simulink model "model_ex2_FUNCIONA_BIEN"  (R2019b)
settings: Solver=VariableStepDiscrete  StartTime=0.0  StopTime=100.0  RelTol=1e-3
values from neighbouring files (symbols this model uses):
  th_0 = input(ask_th)    [simData2.m]
  Ts = Ts * 10.^-3    (= 0.0001)    [simData2.m]
  x_0 = input(ask_x)    [simData2.m]
  y_0 = input(ask_y)    [simData2.m]
undefined symbols (not defined in the file or in its folder): DiscIntNeverNeededParam, sigbuilder_block
libraries: simulink x1
settings Model: Creator=Laura  LastModifiedBy=Laura
settings DataIOCC: SaveFormat=StructureWithTime  ReturnWorkspaceOutputs=off

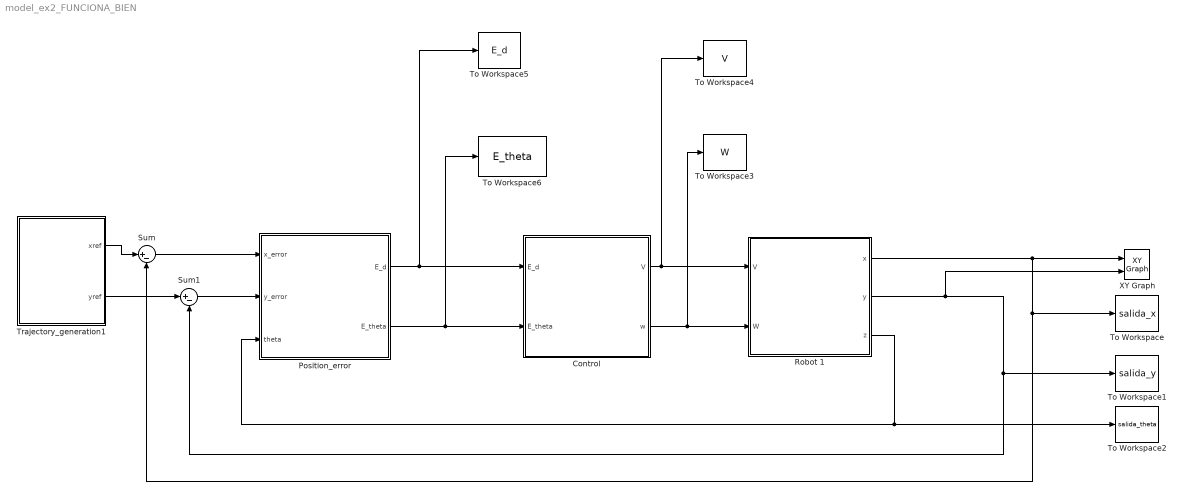
== system model_ex2_FUNCIONA_BIEN ==
  Control : Subsystem
  "Position_error " : Subsystem
  Robot 1 : Subsystem
  Sum : Sum  Inputs=|+-
  Sum1 : Sum  Inputs=|+-
  To Workspace : ToWorkspace  VariableName=salida_x  SaveFormat=Structure With Time  SampleTime=-1
      settings: Save2DSignal=2-D array (concatenate along first dimension)
  To Workspace1 : ToWorkspace  VariableName=salida_y  SaveFormat=Structure With Time  SampleTime=-1
      settings: Save2DSignal=2-D array (concatenate along first dimension)
  To Workspace2 : ToWorkspace  VariableName=salida_theta  SaveFormat=Structure With Time  SampleTime=-1
      settings: Save2DSignal=2-D array (concatenate along first dimension)
  To Workspace3 : ToWorkspace  VariableName=W  SaveFormat=Structure With Time  SampleTime=-1
      settings: Save2DSignal=2-D array (concatenate along first dimension)
  To Workspace4 : ToWorkspace  VariableName=V  SaveFormat=Structure With Time  SampleTime=-1
      settings: Save2DSignal=2-D array (concatenate along first dimension)
  To Workspace5 : ToWorkspace  VariableName=E_d  SaveFormat=Structure With Time  SampleTime=-1
      settings: Save2DSignal=2-D array (concatenate along first dimension)
  To Workspace6 : ToWorkspace  VariableName=E_theta  SaveFormat=Structure With Time  SampleTime=-1
      settings: Save2DSignal=2-D array (concatenate along first dimension)
  Trajectory_generation1 : Subsystem
  XY Graph : simulink/Sinks/XY Graph  xmin=-5  xmax=5  ymin=-5  ymax=5  st=-1
  wires:
  Robot 1/2(y) -> XY Graph/2, Sum1/2, To Workspace1/1
  Control/1(V) -> Robot 1/1("V "), To Workspace4/1
  Control/2(w) -> Robot 1/2("W "), To Workspace3/1
  "Position_error "/1(E_d) -> Control/1(E_d), To Workspace5/1
  Sum/1 -> "Position_error "/1("x_error ")
  "Position_error "/2(E_theta) -> Control/2(E_theta), To Workspace6/1
  Robot 1/1(x) -> XY Graph/1, Sum/2, To Workspace/1
  Robot 1/3(z) -> "Position_error "/3("theta "), To Workspace2/1
  Sum1/1 -> "Position_error "/2("y_error ")
  Trajectory_generation1/1(xref) -> Sum/1
  Trajectory_generation1/2(yref) -> Sum1/1

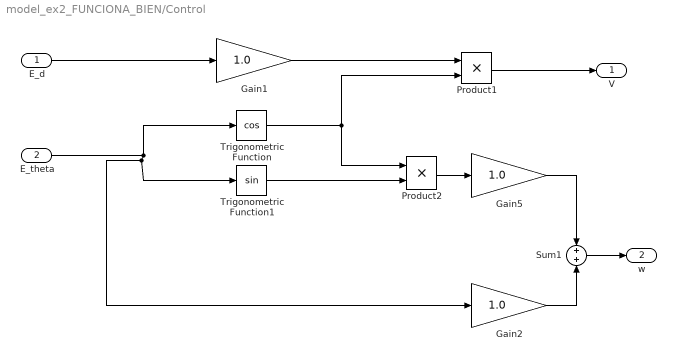
== system model_ex2_FUNCIONA_BIEN/Control ==
  E_d : Inport
  E_theta : Inport  Port=2
  Gain1 : Gain  Gain=1.0
  Gain2 : Gain  Gain=1.0
  Gain5 : Gain  Gain=1.0
  Product1 : Product
  Product2 : Product
  Sum1 : Sum
  Trigonometric Function : Trigonometry  Operator=cos
  Trigonometric Function1 : Trigonometry
  V : Outport  VectorParamsAs1DForOutWhenUnconnected=off
  w : Outport  Port=2  VectorParamsAs1DForOutWhenUnconnected=off
  wires:
  Sum1/1 -> w/1
  Gain2/1 -> Sum1/2
  Gain5/1 -> Sum1/1
  Gain1/1 -> Product1/1
  Product2/1 -> Gain5/1
  Trigonometric Function1/1 -> Product2/2
  Product1/1 -> V/1
  Trigonometric Function/1 -> Product2/1, Product1/2
  E_d/1 -> Gain1/1
  E_theta/1 -> Gain2/1, Trigonometric Function1/1, Trigonometric Function/1

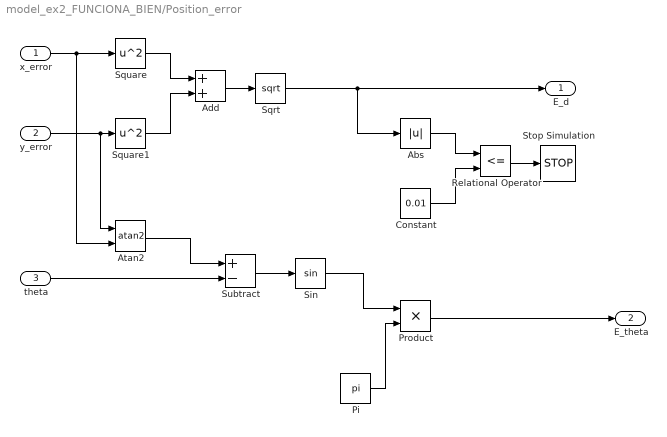
== system model_ex2_FUNCIONA_BIEN/Position_error  ==
  "x_error " : Inport
  "y_error " : Inport  Port=2
  "theta " : Inport  Port=3
  Abs : Abs
  Add : Sum
  Atan2 : Trigonometry  Operator=atan2
  Constant : Constant  Value=0.01
  Pi : Constant  Value=pi  OutDataTypeStr=Inherit: Inherit via back propagation
  Product : Product
  Relational Operator : RelationalOperator  Operator=<=  OutDataTypeStr=boolean  RndMeth=Simplest
  Sin : Trigonometry
  Sqrt : Sqrt  SaturateOnIntegerOverflow=on
  Square : Math  Operator=square  SignedPower=off  SaturateOnIntegerOverflow=on
  Square1 : Math  Operator=square  SignedPower=off  SaturateOnIntegerOverflow=on
  Stop Simulation : Stop
  Subtract : Sum  Inputs=+-
  E_d : Outport
  E_theta : Outport  Port=2
  wires:
  Abs/1 -> Relational Operator/1
  Constant/1 -> Relational Operator/2
  Relational Operator/1 -> Stop Simulation/1
  "x_error "/1 -> Atan2/2, Square/1
  "y_error "/1 -> Atan2/1, Square1/1
  Square/1 -> Add/1
  Square1/1 -> Add/2
  Add/1 -> Sqrt/1
  Atan2/1 -> Subtract/1
  "theta "/1 -> Subtract/2
  Sqrt/1 -> E_d/1, Abs/1
  Subtract/1 -> Sin/1
  Sin/1 -> Product/1
  Pi/1 -> Product/2
  Product/1 -> E_theta/1

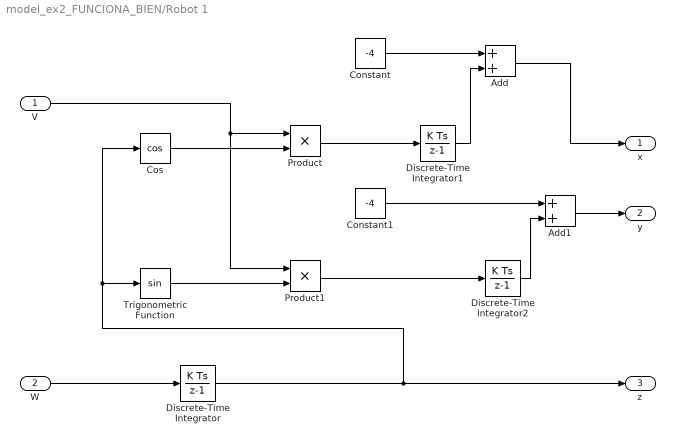
== system model_ex2_FUNCIONA_BIEN/Robot 1 ==
  "V " : Inport
  "W " : Inport  Port=2
  Add : Sum
  Add1 : Sum
  Constant : Constant  Value=-4
  Constant1 : Constant  Value=-4
  Cos : Trigonometry  Operator=cos
  Discrete-Time Integrator : DiscreteIntegrator  InitialCondition=th_0  SampleTime=-1  ICPrevOutput=DiscIntNeverNeededParam  ICPrevScaledInput=DiscIntNeverNeededParam
  Discrete-Time Integrator1 : DiscreteIntegrator  InitialCondition=x_0  SampleTime=-1  ICPrevOutput=DiscIntNeverNeededParam  ICPrevScaledInput=DiscIntNeverNeededParam
  Discrete-Time Integrator2 : DiscreteIntegrator  InitialCondition=y_0  SampleTime=-1  ICPrevOutput=DiscIntNeverNeededParam  ICPrevScaledInput=DiscIntNeverNeededParam
  Product : Product
  Product1 : Product
  Trigonometric Function : Trigonometry
  x : Outport
  y : Outport  Port=2
  z : Outport  Port=3
  wires:
  Product/1 -> Discrete-Time Integrator1/1
  Trigonometric Function/1 -> Product1/2
  Discrete-Time Integrator/1 -> Cos/1, Trigonometric Function/1, z/1
  "W "/1 -> Discrete-Time Integrator/1
  Product1/1 -> Discrete-Time Integrator2/1
  Cos/1 -> Product/2
  "V "/1 -> Product1/1, Product/1
  Discrete-Time Integrator1/1 -> Add/2
  Constant/1 -> Add/1
  Add/1 -> x/1
  Constant1/1 -> Add1/1
  Discrete-Time Integrator2/1 -> Add1/2
  Add1/1 -> y/1

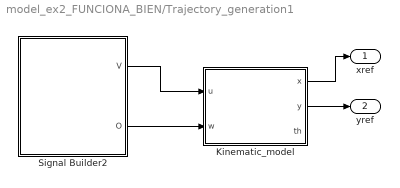
== system model_ex2_FUNCIONA_BIEN/Trajectory_generation1 ==
  Kinematic_model : Subsystem
  Signal Builder2 : Subsystem  Tag=STV Subsys  LoadFcn=sigbuilder_block('load');  StartFcn=sigbuilder_block('start');  StopFcn=sigbuilder_block('stop');  ClipboardFcn=sigbuilder_block('clipboard');  mask(Sigbuilder block){tuvar=[0:10]}
      mask help: Sigbuilder GUI
      mask init:
      | if ~strcmp(get_param(bdroot(gcbh),'SimulationStatus'),'stopped') tuvar = sigbuilder_block('maskInit'); end
      settings: CopyFcn=sigbuilder_block('copy');  DeleteFcn=sigbuilder_block('delete');  ModelCloseFcn=sigbuilder_block('modelClose');  PreSaveFcn=sigbuilder_block('preSave');  PauseFcn=sigbuilder_block('pause')  ContinueFcn=sigbuilder_block('continue')  NameChangeFcn=sigbuilder_block('namechange');  OpenFcn=sigbuilder_block('open',[60 82.4 534.4 508 ]);  CloseFcn=sigbuilder_block('close');
      mask Display: plot(0, 0, 100, 100,[2, 2, 32, 32, 2], [68, 8, 8, 68, 68],[32, 2], [38, 38], [32, 19, 2],[53, 60, 44], [32, 17, 17, 2],[16, 16, 31, 31]);txt = getActiveGroup(gcbh);text(2, 100, txt,'verticalAlignment', 'top');
  xref : Outport  VectorParamsAs1DForOutWhenUnconnected=off
  yref : Outport  Port=2  VectorParamsAs1DForOutWhenUnconnected=off
  wires:
  Signal Builder2/1(V) -> Kinematic_model/1(u)
  Signal Builder2/2(O) -> Kinematic_model/2(w)
  Kinematic_model/1(x) -> xref/1
  Kinematic_model/2(y) -> yref/1

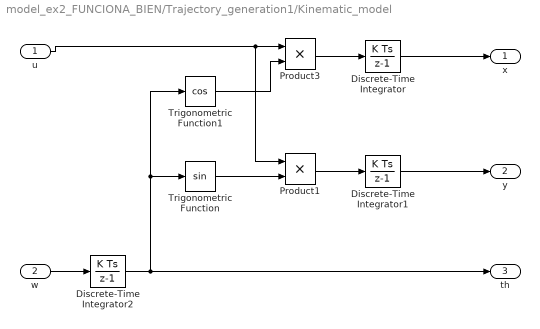
== system model_ex2_FUNCIONA_BIEN/Trajectory_generation1/Kinematic_model ==
  u : Inport
  w : Inport  Port=2
  Discrete-Time Integrator : DiscreteIntegrator  InitialCondition=x_0  SampleTime=Ts  ICPrevOutput=DiscIntNeverNeededParam  ICPrevScaledInput=DiscIntNeverNeededParam
  Discrete-Time Integrator1 : DiscreteIntegrator  InitialCondition=y_0  SampleTime=Ts  ICPrevOutput=DiscIntNeverNeededParam  ICPrevScaledInput=DiscIntNeverNeededParam
  Discrete-Time Integrator2 : DiscreteIntegrator  InitialCondition=th_0  SampleTime=Ts  ICPrevOutput=DiscIntNeverNeededParam  ICPrevScaledInput=DiscIntNeverNeededParam
  Product1 : Product
  Product3 : Product
  Trigonometric Function : Trigonometry
  Trigonometric Function1 : Trigonometry  Operator=cos
  x : Outport  VectorParamsAs1DForOutWhenUnconnected=off
  y : Outport  Port=2  VectorParamsAs1DForOutWhenUnconnected=off
  th : Outport  Port=3  VectorParamsAs1DForOutWhenUnconnected=off
  wires:
  Discrete-Time Integrator2/1 -> Trigonometric Function1/1, Trigonometric Function/1, th/1
  Product1/1 -> Discrete-Time Integrator1/1
  Product3/1 -> Discrete-Time Integrator/1
  w/1 -> Discrete-Time Integrator2/1
  Trigonometric Function/1 -> Product1/2
  u/1 -> Product1/1, Product3/1
  Trigonometric Function1/1 -> Product3/2
  Discrete-Time Integrator1/1 -> y/1
  Discrete-Time Integrator/1 -> x/1

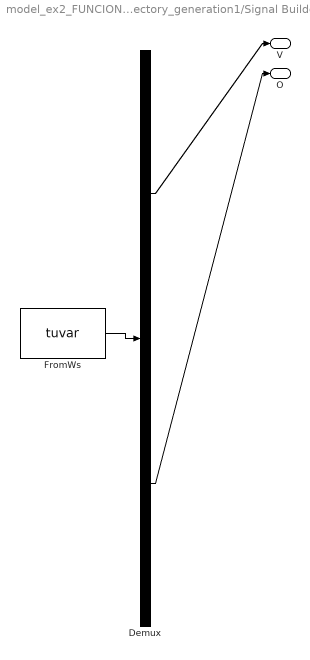
== system model_ex2_FUNCIONA_BIEN/Trajectory_generation1/Signal Builder2 ==
  Demux : Demux  Tag=STV Demux  Outputs=2
  FromWs : FromWorkspace  Tag=STV FromWs  VariableName=tuvar  SampleTime=0
      SigBuilderData=|
      | common.afterFinalStr = 'Extrapolate'
      | common.sampleTime = '0'
      | dataSet.timeRange = [0 115]
      | dataSet.name = 'Group 1'
      | sbobj.Groups.Name = 'Group 1'
      | sbobj.Groups.Signals(1).Name = 'V'
      | sbobj.Groups.Signals(1).XData = [0 87 87 115]
      | sbobj.Groups.Signals(1).YData = [0.25 0.25 0 0]
      | sbobj.Groups.Signals(2).Name = 'O'
      | sbobj.Groups.Signals(2).XData = [0 12 12 30.849 30.849 55.981 55.981 74.83 74.83 99.962 115]
      | sbobj.Groups.Signals(2).YData = [0 0 0.25 0.25 -0.25 -0.25 0.25 0.25 0 0 0]
      | sbobj.Groups.TimeRange = [0 115]
  V : Outport  Tag=STV Outport  VectorParamsAs1DForOutWhenUnconnected=off
  O : Outport  Tag=STV Outport  Port=2  VectorParamsAs1DForOutWhenUnconnected=off
  wires:
  FromWs/1 -> Demux/1
  Demux/1 -> V/1
  Demux/2 -> O/1
